simulink model "Appl_VentAdj_CtrlModel"  (R2018b)
settings: configuration reference "CodeConfig_10_ms" (kept outside this file)
undefined symbols (not defined in the file): D_VENT_LVL_1_PRECENT, D_VENT_LVL_2_PRECENT, D_VENT_LVL_3_PRECENT, FALSE, TRUE
libraries: DareLib x72, simulink x1
(part 3 of 4)

== stateflow chart Appl_VentAdj_CtrlModel/LogicCtrl/LocalAdjustCtrl/LimitDeal/TimeoutFunction1/Timeout ==
  state Ts = D_HAL_GET_CUR_MS_TS [function]
  state OutTs = TimeDiffTs(lastTs,Ts) [function]
  state TimeCountStatus
    state TimeoutSts
      en:
      Level = InLevel;
      du:
      Level = InLevel;
      ex:
      Timer = 0;
    state Init
      en:
      Level = InLevel;
      Timer = D_HAL_GET_CUR_MS_TS();
      du:
      Level = InLevel;
      ex:
      Timer = D_HAL_GET_CUR_MS_TS();
    (default) -> Init
    Init -> TimeoutSts [order 1] : [TimeDiffTs(Timer,D_HAL_GET_CUR_MS_TS()) >= MaxTime]
        | /TimeoutFlag = TRUE;
    TimeoutSts -> Init : [hasChangedFrom(InLevel,enVentLvlSts.EN_VENT_LVL_OFF)]
    Init -> Init [order 2] : [hasChangedFrom(InLevel,enVentLvlSts.EN_VENT_LVL_OFF)]
  state Default
    en:
    Level = InLevel;
    du:
    Level = InLevel;
  (default) -> Default
  Default -> TimeCountStatus : /*有超时配置
      | && 启动加热&&有时间值 */
      | [TRUE == TimeoutPrm ...
      | && enVentLvlSts.EN_VENT_LVL_OFF != InLevel ...
      | && 0 != MaxTime]
  TimeCountStatus -> Default : /*无超时配置*/
      | [TRUE != TimeoutPrm || 0 == MaxTime]
      | /TimeoutFlag = FALSE;
  data: Ts function_output; lastTs function_input; Ts function_input; OutTs function_output; TimeoutPrm input uint8; TimeoutFlag output uint8; FALSE parameter; TRUE parameter; InLevel input Enum: enVentLvlSts; MaxTime input uint32; Timer local uint32; Level output Enum: enVentLvlSts

== stateflow chart Appl_VentAdj_CtrlModel/UpDataInputInfo/InputSignalProcess/HeatMessage/HeatMessage ==
  state VenSts = OppositeMessageDeal(CarTypeCfg,RemoteModeFlag,HMI_Message,Tbox_Message,HeatCfg) [function]
  state VenSts = OppositeMessageDeal1(CarTypeCfg,RemoteModeFlag,HMI_Message,Tbox_Message,HeatCfg) [function]
  state VenSts = OppositeMessageDeal2(CarTypeCfg,RemoteModeFlag,HMI_Message,Tbox_Message,HeatCfg) [function]
  state run
    du:
    DriverHeatValid = OppositeMessageDeal(VentAdj_CarType,VentAdj_RemoteModeFlag,VentAdj_Driver_HMI_HeatMsg,VentAdj_Driver_Tbox_HeatMsg,VentAdj_DrHeatFlg);
    PassengerHeatValid = OppositeMessageDeal1(VentAdj_CarType,VentAdj_RemoteModeFlag,VentAdj_Passenger_HMI_HeatMsg,VentAdj_Passenger_Tbox_HeatMsg,VentAdj_PaHeatFlg);
    ThirdHeatValid = OppositeMessageDeal2(VentAdj_CarType,VentAdj_RemoteModeFlag,VentAdj_Third_HMI_HeatMsg,VentAdj_Third_Tbox_HeatMsg,VentAdj_3rdHeatFlg);
  (default) -> run
  data: CarTypeCfg function_input; RemoteModeFlag function_input; HMI_Message function_input; Tbox_Message function_input; VenSts function_output; HeatCfg function_input; CarTypeCfg function_input; RemoteModeFlag function_input; HMI_Message function_input; Tbox_Message function_input; VenSts function_output; HeatCfg function_input; CarTypeCfg function_input; RemoteModeFlag function_input; HMI_Message function_input; Tbox_Message function_input; VenSts function_output; HeatCfg function_input; DriverHeatValid output uint8; PassengerHeatValid output uint8; ThirdHeatValid output uint8; VentAdj_CarType input; VentAdj_Driver_HMI_HeatMsg input; VentAdj_Driver_Tbox_HeatMsg input; VentAdj_Passenger_HMI_HeatMsg input; VentAdj_Passenger_Tbox_HeatMsg input; VentAdj_Third_HMI_HeatMsg input; VentAdj_Third_Tbox_HeatMsg input; VentAdj_RemoteModeFlag input; VentAdj_DrHeatFlg input; VentAdj_PaHeatFlg input; VentAdj_3rdHeatFlg input

== stateflow chart Appl_VentAdj_CtrlModel/UpDataInputInfo/InputSignalProcess/HeatMessage/HeatMessage/OppositeMessageDeal1/OppositeMessageDeal ==
  state HMIMessageDeal [parallel]
    settings: executionOrder=1
    state HMIValid
      en:
      TempHMI = TRUE;
    state HMIInit
      en:
      TempHMI = FALSE;
    (default) -> HMIInit
    HMIInit -> HMIValid : /*档位请求有效*/
        | [(enProjectType.EN_PROJECT_BM400 != CarTypeCfg && (0x1 == HMI_Message || 0x2 == HMI_Message || 0x3 == HMI_Message || 0x5 == HMI_Message)) ...
        | || (enProjectType.EN_PROJECT_BM400 == CarTypeCfg && (0x2 == HMI_Message || 0x3 == HMI_Message || 0x4 == HMI_Message))]
    HMIValid -> HMIInit : /*HMI报文关闭*/
        | [(enProjectType.EN_PROJECT_BM400 != CarTypeCfg && 0x1 != HMI_Message && 0x2 != HMI_Message && 0x3 != HMI_Message&& 0x5 != HMI_Message) ...
        | || (enProjectType.EN_PROJECT_BM400 == CarTypeCfg && 0x2 != HMI_Message && 0x3 != HMI_Message && 0x4 != HMI_Message)]
  state TboxMessageDeal [parallel]
    settings: executionOrder=2
    state TboxValid
      en:
      TempTbox = TRUE;
    state TboxInit
      en:
      TempTbox = FALSE;
    (default) -> TboxMessageDeal.TboxInit
    TboxMessageDeal.TboxInit -> TboxMessageDeal.TboxValid : /*档位请求有效*/
        | [(TRUE == RemoteModeFlag) && (0x1 == Tbox_Message ...
        | || 0x2 == Tbox_Message ...
        | || 0x3 == Tbox_Message)]
    TboxMessageDeal.TboxValid -> TboxMessageDeal.TboxInit : /*Tbox报文关闭*/
        | [0x0 == Tbox_Message || FALSE == RemoteModeFlag]
  state VenStatus [parallel]
    settings: executionOrder=3
    state TboxValid
      en:
      VenSts = TRUE;
    state TboxInit
      en:
      VenSts = FALSE;
    (default) -> VenStatus.TboxInit
    VenStatus.TboxInit -> VenStatus.TboxValid : /* 档位请求有效 且加热配置 */
        | [(TRUE == TempHMI ...
        | || TRUE == TempTbox) && HeatCfg == TRUE]
    VenStatus.TboxValid -> VenStatus.TboxInit : /* 档位请求无效 或加热无配置 */
        | [(FALSE == TempHMI ...
        | && FALSE == TempTbox) || HeatCfg == FALSE]
  data: CarTypeCfg input Enum: enProjectType; RemoteModeFlag input uint8; HMI_Message input uint8; Tbox_Message input uint8; VenSts output uint8; TempHMI local uint8; TRUE parameter; FALSE parameter; TempTbox local uint8; HeatCfg input uint8

== stateflow chart Appl_VentAdj_CtrlModel/LogicCtrl/LocalAdjustCtrl/LimitDeal/DiagnoseFunction1/Diagnose ==
  state Diagnose
    (default) -> (junction 3)
    Diagnose -> (junction 3)
    (junction 3) -> (junction 6)
    (junction 6) -> (junction 8) [order 1] : /* 无诊断指令 */
        | [0 == DiagCommand || DiagCommand > (enVentLvlSts.EN_VENT_LVL_3 + 1)]
    (junction 6) -> (junction 14) [order 2] : {Level = DiagCommand - 1;
        | Type = enVentType.EN_VENT_TYPE_DIAG;}
    (junction 8) -> (junction 10) : {Level = InLevel;
        | Type = CurrentType;}
    (junction 10) -> (junction 14)
    (junction 14) -> (junction 17)
  (default) -> Diagnose
  data: DiagCommand input uint8; InLevel input Enum: enVentLvlSts; CurrentType input Enum: enVentType; Level output Enum: enVentLvlSts; Type output Enum: enVentType

== stateflow chart Appl_VentAdj_CtrlModel/LogicCtrl/LocalAdjustCtrl/LimitDeal/DiagnoseFunction2/Diagnose ==
  state Diagnose
    (default) -> (junction 3)
    Diagnose -> (junction 3)
    (junction 3) -> (junction 6)
    (junction 6) -> (junction 8) [order 1] : /* 无诊断指令 */
        | [0 == DiagCommand || DiagCommand > (enVentLvlSts.EN_VENT_LVL_3 + 1)]
    (junction 6) -> (junction 14) [order 2] : {Level = DiagCommand - 1;
        | Type = enVentType.EN_VENT_TYPE_DIAG;}
    (junction 8) -> (junction 10) : {Level = InLevel;
        | Type = CurrentType;}
    (junction 10) -> (junction 14)
    (junction 14) -> (junction 17)
  (default) -> Diagnose
  data: DiagCommand input uint8; InLevel input Enum: enVentLvlSts; CurrentType input Enum: enVentType; Level output Enum: enVentLvlSts; Type output Enum: enVentType

== stateflow chart Appl_VentAdj_CtrlModel/LogicCtrl/LocalAdjustCtrl/LimitDeal/StopFunction1/StopFunction ==
  state ValidSts
    en:
    StopReason = enVentStopReason.EN_VENT_STOP_R_TIME;
    du:
    StopReason = enVentStopReason.EN_VENT_STOP_R_TIME;
  state Default
    en:
    du:
    StopReason = ComStop;
    du:
    StopReason = ComStop;
  (default) -> Default
  Default -> ValidSts : /*无通用限制
      | &&超时限制有效*/
      | [enVentStopReason.EN_VENT_STOP_R_NONE == ComStop ...
      | && TRUE  == Timeout]
  ValidSts -> Default : /*无超时限制*/
      | [FALSE  == Timeout]
  data: FALSE parameter; StopReason output Enum: enVentStopReason; Timeout input uint8; ComStop input Enum: enVentStopReason; TRUE parameter

== stateflow chart Appl_VentAdj_CtrlModel/LogicCtrl/LocalAdjustCtrl/LimitDeal/StopFunction2/StopFunction ==
  state ValidSts
    en:
    StopReason = enVentStopReason.EN_VENT_STOP_R_TIME;
    du:
    StopReason = enVentStopReason.EN_VENT_STOP_R_TIME;
  state Default
    en:
    du:
    StopReason = ComStop;
    du:
    StopReason = ComStop;
  (default) -> Default
  Default -> ValidSts : /*无通用限制
      | &&超时限制有效*/
      | [enVentStopReason.EN_VENT_STOP_R_NONE == ComStop ...
      | && TRUE  == Timeout]
  ValidSts -> Default : /*无超时限制*/
      | [FALSE  == Timeout]
  data: FALSE parameter; StopReason output Enum: enVentStopReason; Timeout input uint8; ComStop input Enum: enVentStopReason; TRUE parameter

== stateflow chart Appl_VentAdj_CtrlModel/LogicCtrl/LocalAdjustCtrl/LimitDeal/StopFunction/StopFunction ==
  state ValidSts
    en:
    StopReason = enVentStopReason.EN_VENT_STOP_R_TIME;
    du:
    StopReason = enVentStopReason.EN_VENT_STOP_R_TIME;
  state Default
    en:
    du:
    StopReason = ComStop;
    du:
    StopReason = ComStop;
  (default) -> Default
  Default -> ValidSts : /*无通用限制
      | &&超时限制有效*/
      | [enVentStopReason.EN_VENT_STOP_R_NONE == ComStop ...
      | && TRUE  == Timeout]
  ValidSts -> Default : /*无超时限制*/
      | [FALSE  == Timeout]
  data: FALSE parameter; StopReason output Enum: enVentStopReason; Timeout input uint8; ComStop input Enum: enVentStopReason; TRUE parameter

== stateflow chart Appl_VentAdj_CtrlModel/LogicCtrl/LocalAdjustCtrl/LimitDeal/DiagnoseFunction/Diagnose ==
  state Diagnose
    (default) -> (junction 3)
    Diagnose -> (junction 3)
    (junction 3) -> (junction 6)
    (junction 6) -> (junction 8) [order 1] : /* 无诊断指令 */
        | [0 == DiagCommand || DiagCommand > (enVentLvlSts.EN_VENT_LVL_3 + 1)]
    (junction 6) -> (junction 14) [order 2] : {Level = DiagCommand - 1;
        | Type = enVentType.EN_VENT_TYPE_DIAG;}
    (junction 8) -> (junction 10) : {Level = InLevel;
        | Type = CurrentType;}
    (junction 10) -> (junction 14)
    (junction 14) -> (junction 17)
  (default) -> Diagnose
  data: DiagCommand input uint8; InLevel input Enum: enVentLvlSts; CurrentType input Enum: enVentType; Level output Enum: enVentLvlSts; Type output Enum: enVentType

== stateflow chart Appl_VentAdj_CtrlModel/LogicCtrl/LocalAdjustCtrl/OutputDeal ==
  state CANOutputDeal [parallel]
    settings: executionOrder=1
    state ProjectP20
      en:
      /*Initial Value(Hex)初始值:0x0*/
      OutDrCANVentLevel = 0;
      OutPaCANVentLevel = 0;
      Out3rdCANVentLevel = 0;
      state Drv [parallel]
        settings: executionOrder=1
        state Run
          en:
          OutDrCANVentLevel = DiagDrVentLevel;
          LocalDrRunState = TRUE;
          du:
          OutDrCANVentLevel = DiagDrVentLevel;
          LocalDrRunState = TRUE;
        state Init
          en:
          LocalDrRunState = FALSE;
        (default) -> CANOutputDeal.ProjectP20.Drv.Init
        CANOutputDeal.ProjectP20.Drv.Init -> CANOutputDeal.ProjectP20.Drv.Run : /* 主驾通风指令 */
            | [enVentLvlSts.EN_VENT_LVL_OFF != DiagDrVentLevel]
        CANOutputDeal.ProjectP20.Drv.Run -> CANOutputDeal.ProjectP20.Drv.Init : /* 主驾通风无指令 */
            | [enVentLvlSts.EN_VENT_LVL_OFF == DiagDrVentLevel]
      state Pas [parallel]
        settings: executionOrder=2
        state Run
          en:
          OutPaCANVentLevel = DiagPaVentLevel;
          LocalPaRunState = TRUE;
          du:
          OutPaCANVentLevel = DiagPaVentLevel;
          LocalPaRunState = TRUE;
        state Init
          en:
          LocalPaRunState = FALSE;
        (default) -> CANOutputDeal.ProjectP20.Pas.Init
        CANOutputDeal.ProjectP20.Pas.Run -> CANOutputDeal.ProjectP20.Pas.Init : /* 副驾通风无指令 */
            | [enVentLvlSts.EN_VENT_LVL_OFF == DiagPaVentLevel]
        CANOutputDeal.ProjectP20.Pas.Init -> CANOutputDeal.ProjectP20.Pas.Run : /* 副驾通风指令 */
            | [enVentLvlSts.EN_VENT_LVL_OFF != DiagPaVentLevel]
      state Treble [parallel]
        settings: executionOrder=3
        state Init
          en:
          Local3rdRunState = FALSE;
        state Run
          en:
          Out3rdCANVentLevel = Diag3rdVentLevel;
          Local3rdRunState = TRUE;
          du:
          Out3rdCANVentLevel = Diag3rdVentLevel;
          Local3rdRunState = TRUE;
        (default) -> CANOutputDeal.ProjectP20.Treble.Init
        CANOutputDeal.ProjectP20.Treble.Init -> CANOutputDeal.ProjectP20.Treble.Run : /* 三排通风无指令 */
            | [enVentLvlSts.EN_VENT_LVL_OFF != Diag3rdVentLevel]
        CANOutputDeal.ProjectP20.Treble.Run -> CANOutputDeal.ProjectP20.Treble.Init : /* 三排通风无指令 */
            | [enVentLvlSts.EN_VENT_LVL_OFF == Diag3rdVentLevel]
    state Default
      en:
      OutDrCANVentLevel = DiagDrVentLevel;
      OutPaCANVentLevel = DiagPaVentLevel;
      Out3rdCANVentLevel = Diag3rdVentLevel;
      OutDrRunState = FALSE;
      OutPaRunState = FALSE;
      Out3rdRunState = FALSE;
      LocalDrRunState = FALSE;
      LocalDrRunState = FALSE;
      LocalDrRunState = FALSE;
      du:
      OutDrCANVentLevel = DiagDrVentLevel;
      OutPaCANVentLevel = DiagPaVentLevel;
      Out3rdCANVentLevel = Diag3rdVentLevel;
      OutDrRunState = FALSE;
      OutPaRunState = FALSE;
      Out3rdRunState = FALSE;
      LocalDrRunState = FALSE;
      LocalDrRunState = FALSE;
      LocalDrRunState = FALSE;
    (default) -> Default
    Default -> ProjectP20 : /* P20的车型 */
        | [enProjectType.EN_PROJECT_P20 == CarTypeCfg]
    ProjectP20 -> Default : /* 非P20车型 */
        | [enProjectType.EN_PROJECT_P20 != CarTypeCfg]
  state DrvErr [parallel]
    settings: executionOrder=2
    state FalseSts
      en:
      OutDrRunState = LocalDrRunState;
      du:
      OutDrRunState = LocalDrRunState;
    state SuccSts
      en:
      OutDrRunState = 2;
      du:
      OutDrRunState = 2;
    (default) -> DrvErr.FalseSts
    DrvErr.FalseSts -> DrvErr.SuccSts : /* 无指令 且存在故障 */
        | [LocalDrRunState == FALSE ...
        | && VentAdj_DriverCmdFaultSts4DTC != FALSE]
    DrvErr.SuccSts -> DrvErr.FalseSts : /*无故障 或RUN状态 */
        | [LocalDrRunState == TRUE ...
        | || VentAdj_DriverCmdFaultSts4DTC ==  FALSE]
  state AcquireDuty [parallel]
    en:
    DrAimDuty = DutyFunction(DiagDrVentLevel);
    PaAimDuty = DutyFunction(DiagPaVentLevel);
    ThirdAimDuty = DutyFunction(Diag3rdVentLevel);
    du:
    DrAimDuty = DutyFunction(DiagDrVentLevel);
    PaAimDuty = DutyFunction(DiagPaVentLevel);
    ThirdAimDuty = DutyFunction(Diag3rdVentLevel);
    settings: executionOrder=5
  state AimDuty = DutyFunction(AimLevel) [function]
  state PasErr [parallel]
    settings: executionOrder=3
    state FalseSts
      en:
      OutPaRunState = LocalPaRunState;
      du:
      OutPaRunState = LocalPaRunState;
    state SuccSts
      en:
      OutPaRunState = 2;
      du:
      OutPaRunState = 2;
    (default) -> PasErr.FalseSts
    PasErr.FalseSts -> PasErr.SuccSts : /* 无指令 且存在故障 */
        | [LocalPaRunState == FALSE ...
        | && VentAdj_PasCmdFaultSts4DTC != FALSE]
    PasErr.SuccSts -> PasErr.FalseSts : /*无故障 或RUN状态 */
        | [LocalPaRunState == TRUE ...
        | || VentAdj_PasCmdFaultSts4DTC == FALSE]
  state TrebleErr [parallel]
    settings: executionOrder=4
    state FalseSts
      en:
      Out3rdRunState = Local3rdRunState;
      du:
      Out3rdRunState = Local3rdRunState;
    state SuccSts
      en:
      Out3rdRunState = 2;
      du:
      Out3rdRunState = 2;
    (default) -> TrebleErr.FalseSts
    TrebleErr.FalseSts -> TrebleErr.SuccSts : /* 无指令 且存在故障 */
        | [Local3rdRunState == FALSE ...
        | && VentAdj_ThirdCmdFaultSts4DTC != FALSE]
    TrebleErr.SuccSts -> TrebleErr.FalseSts : /*无故障 或RUN状态 */
        | [Local3rdRunState == TRUE ...
        | || VentAdj_ThirdCmdFaultSts4DTC == FALSE]
  data: AimLevel function_input; AimDuty function_output; OutDrCANVentLevel output Enum: enVentLvlSts; OutPaCANVentLevel output Enum: enVentLvlSts; Out3rdCANVentLevel output Enum: enVentLvlSts; CarTypeCfg input; DiagDrVentLevel input; DiagPaVentLevel input; Diag3rdVentLevel input; FALSE parameter; OutDrRunState output uint8; OutPaRunState output uint8; Out3rdRunState output uint8; TRUE parameter; DrAimDuty output uint8; PaAimDuty output uint8; ThirdAimDuty output uint8; LocalDrRunState local uint8; LocalPaRunState local uint8; Local3rdRunState local uint8; VentAdj_DriverCmdFaultSts4DTC input; VentAdj_PasCmdFaultSts4DTC input; VentAdj_ThirdCmdFaultSts4DTC input

== stateflow chart Appl_VentAdj_CtrlModel/LogicCtrl/LocalAdjustCtrl/OutputDeal/DutyFunction/Duty ==
  (default) -> (junction 3)
  (junction 3) -> (junction 5) : {AimDuty = 100;}
  (junction 5) -> (junction 7) [order 1] : /* 通风1档 */
      | [enVentLvlSts.EN_VENT_LVL_1 == AimLevel]
  (junction 5) -> (junction 11) [order 2]
  (junction 7) -> (junction 9) : {AimDuty = D_VENT_LVL_1_PRECENT;}
  (junction 9) -> (junction 11)
  (junction 11) -> (junction 14)
  (junction 14) -> (junction 16) [order 1] : /* 通风2档 */
      | [enVentLvlSts.EN_VENT_LVL_2 == AimLevel]
  (junction 14) -> (junction 20) [order 2]
  (junction 16) -> (junction 18) : {AimDuty = D_VENT_LVL_2_PRECENT;}
  (junction 18) -> (junction 20)
  (junction 20) -> (junction 23)
  (junction 23) -> (junction 25) [order 1] : /* 通风3档 */
      | [enVentLvlSts.EN_VENT_LVL_3 == AimLevel]
  (junction 23) -> (junction 29) [order 2]
  (junction 25) -> (junction 27) : {AimDuty = D_VENT_LVL_3_PRECENT;}
  (junction 27) -> (junction 29)
  (junction 29) -> (junction 35)
  data: AimDuty output uint8; AimLevel input Enum: enVentLvlSts; D_VENT_LVL_1_PRECENT parameter; D_VENT_LVL_2_PRECENT parameter; D_VENT_LVL_3_PRECENT parameter

== stateflow chart Appl_VentAdj_CtrlModel/LogicCtrl/LocalAdjustCtrl/VentLevelDeal/VentRunTypeFunction/VentRunType ==
  (default) -> (junction 82)
  (junction 82) -> (junction 84) : {OutLevel = PreLevel;}
  (junction 84) -> (junction 86) [order 1] : /* 有效档位 */
      | [InLevel <= enVentLvlSts.EN_VENT_LVL_3]
  (junction 84) -> (junction 90) [order 2]
  (junction 86) -> (junction 88) : {RunType = InType;
      | OutLevel = InLevel;}
  (junction 88) -> (junction 90)
  (junction 90) -> (junction 93)
  (junction 93) -> (junction 95) [order 1] : /* 通风档位关闭 */
      | [InLevel == enVentLvlSts.EN_VENT_LVL_OFF]
  (junction 93) -> (junction 99) [order 2]
  (junction 95) -> (junction 97) : {RunType = enVentType.EN_VENT_TYPE_NONE;}
  (junction 97) -> (junction 99)
  (junction 99) -> (junction 102)
  data: InLevel input uint8; PreLevel input Enum: enVentLvlSts; InType input Enum: enVentType; RunType output Enum: enVentType; OutLevel output Enum: enVentLvlSts

== stateflow chart Appl_VentAdj_CtrlModel/LogicCtrl/LocalAdjustCtrl/LimitDeal/TimeoutFunction1/Timeout/TimeDiffTs/Chart ==
  (default) -> (junction 3)
  (junction 3) -> (junction 5)
  (junction 5) -> (junction 7) [order 1] : /* 入参比当前大 */
      | [lastTs > Ts]
  (junction 5) -> (junction 13) [order 2] : {OutTs = Ts - lastTs;}
  (junction 7) -> (junction 11) : {OutTs = 0xFFFFFFFF - lastTs + Ts +1;}
  (junction 11) -> (junction 13)
  (junction 13) -> (junction 17)
  data: lastTs input uint32; Ts input uint32; OutTs output uint32

== stateflow chart Appl_VentAdj_CtrlModel/UpDataInputInfo/InputSignalProcess/HeatMessage/HeatMessage/OppositeMessageDeal/OppositeMessageDeal ==
  state HMIMessageDeal [parallel]
    settings: executionOrder=1
    state HMIValid
      en:
      TempHMI = TRUE;
    state HMIInit
      en:
      TempHMI = FALSE;
    (default) -> HMIInit
    HMIInit -> HMIValid : /*档位请求有效*/
        | [(enProjectType.EN_PROJECT_BM400 != CarTypeCfg && (0x1 == HMI_Message || 0x2 == HMI_Message || 0x3 == HMI_Message || 0x5 == HMI_Message)) ...
        | || (enProjectType.EN_PROJECT_BM400 == CarTypeCfg && (0x2 == HMI_Message || 0x3 == HMI_Message || 0x4 == HMI_Message))]
    HMIValid -> HMIInit : /*HMI报文关闭*/
        | [(enProjectType.EN_PROJECT_BM400 != CarTypeCfg && 0x1 != HMI_Message && 0x2 != HMI_Message && 0x3 != HMI_Message&& 0x5 != HMI_Message) ...
        | || (enProjectType.EN_PROJECT_BM400 == CarTypeCfg && 0x2 != HMI_Message && 0x3 != HMI_Message && 0x4 != HMI_Message)]
  state TboxMessageDeal [parallel]
    settings: executionOrder=2
    state TboxValid
      en:
      TempTbox = TRUE;
    state TboxInit
      en:
      TempTbox = FALSE;
    (default) -> TboxMessageDeal.TboxInit
    TboxMessageDeal.TboxInit -> TboxMessageDeal.TboxValid : /*档位请求有效*/
        | [(TRUE == RemoteModeFlag) && (0x1 == Tbox_Message ...
        | || 0x2 == Tbox_Message ...
        | || 0x3 == Tbox_Message)]
    TboxMessageDeal.TboxValid -> TboxMessageDeal.TboxInit : /*Tbox报文关闭*/
        | [0x0 == Tbox_Message || FALSE == RemoteModeFlag]
  state VenStatus [parallel]
    settings: executionOrder=3
    state TboxValid
      en:
      VenSts = TRUE;
    state TboxInit
      en:
      VenSts = FALSE;
    (default) -> VenStatus.TboxInit
    VenStatus.TboxInit -> VenStatus.TboxValid : /* 档位请求有效 且加热配置 */
        | [(TRUE == TempHMI ...
        | || TRUE == TempTbox) && HeatCfg == TRUE]
    VenStatus.TboxValid -> VenStatus.TboxInit : /* 档位请求无效 或加热无配置 */
        | [(FALSE == TempHMI ...
        | && FALSE == TempTbox) || HeatCfg == FALSE]
  data: CarTypeCfg input Enum: enProjectType; RemoteModeFlag input uint8; HMI_Message input uint8; Tbox_Message input uint8; VenSts output uint8; TempHMI local uint8; TRUE parameter; FALSE parameter; TempTbox local uint8; HeatCfg input uint8

== stateflow chart Appl_VentAdj_CtrlModel/LogicCtrl/LocalAdjustCtrl/LimitDeal/TimeoutFunction2/Timeout ==
  state Ts = D_HAL_GET_CUR_MS_TS [function]
  state OutTs = TimeDiffTs(lastTs,Ts) [function]
  state TimeCountStatus
    state TimeoutSts
      en:
      Level = InLevel;
      du:
      Level = InLevel;
      ex:
      Timer = 0;
    state Init
      en:
      Level = InLevel;
      Timer = D_HAL_GET_CUR_MS_TS();
      du:
      Level = InLevel;
      ex:
      Timer = D_HAL_GET_CUR_MS_TS();
    (default) -> Init
    Init -> TimeoutSts [order 1] : [TimeDiffTs(Timer,D_HAL_GET_CUR_MS_TS()) >= MaxTime]
        | /TimeoutFlag = TRUE;
    TimeoutSts -> Init : [hasChangedFrom(InLevel,enVentLvlSts.EN_VENT_LVL_OFF)]
    Init -> Init [order 2] : [hasChangedFrom(InLevel,enVentLvlSts.EN_VENT_LVL_OFF)]
  state Default
    en:
    Level = InLevel;
    du:
    Level = InLevel;
  (default) -> Default
  Default -> TimeCountStatus : /*有超时配置
      | && 启动加热&&有时间值 */
      | [TRUE == TimeoutPrm ...
      | && enVentLvlSts.EN_VENT_LVL_OFF != InLevel ...
      | && 0 != MaxTime]
  TimeCountStatus -> Default : /*无超时配置*/
      | [TRUE != TimeoutPrm || 0 == MaxTime]
      | /TimeoutFlag = FALSE;
  data: Ts function_output; lastTs function_input; Ts function_input; OutTs function_output; TimeoutPrm input uint8; TimeoutFlag output uint8; FALSE parameter; TRUE parameter; InLevel input Enum: enVentLvlSts; MaxTime input uint32; Timer local uint32; Level output Enum: enVentLvlSts

== stateflow chart Appl_VentAdj_CtrlModel/LogicCtrl/LocalAdjustCtrl/LimitDeal/TimeoutFunction2/Timeout/TimeDiffTs/Chart ==
  (default) -> (junction 3)
  (junction 3) -> (junction 5)
  (junction 5) -> (junction 7) [order 1] : /* 入参比当前大 */
      | [lastTs > Ts]
  (junction 5) -> (junction 13) [order 2] : {OutTs = Ts - lastTs;}
  (junction 7) -> (junction 11) : {OutTs = 0xFFFFFFFF - lastTs + Ts +1;}
  (junction 11) -> (junction 13)
  (junction 13) -> (junction 17)
  data: lastTs input uint32; Ts input uint32; OutTs output uint32

== stateflow chart Appl_VentAdj_CtrlModel/LogicCtrl/LocalAdjustCtrl/LimitDeal/LevelLimitFunction/LevelLimit ==
  state Default
    en:
    Level = enVentLvlSts.EN_VENT_LVL_OFF;
  state Run
    en:
    Level = OriginalLevel;
    du:
    Level = OriginalLevel;
  state ForbidStatus
    en:
    Level = enVentLvlSts.EN_VENT_LVL_OFF;
    ex:
    StopReason = enVentStopReason.EN_VENT_STOP_R_NONE;
    (default) -> (junction 74)
    ForbidStatus -> (junction 74) [order 1]
    (junction 74) -> (junction 46) [order 1] : /*存在故障*/
        | [enVentCmdFault.EN_VENT_FAULT_NONE != Error]
    (junction 74) -> (junction 71) [order 2]
    (junction 46) -> (junction 60) : {StopReason = enVentStopReason.EN_VENT_STOP_R_FAULT;}
    (junction 60) -> (junction 71)
    (junction 71) -> (junction 70)
    (junction 70) -> (junction 43) [order 1] : /*互斥命令有效*/
        | [TRUE == OppositeCmd]
    (junction 70) -> (junction 54) [order 2]
    (junction 43) -> (junction 49) : {StopReason = enVentStopReason.EN_VENT_STOP_R_CMD;}
    (junction 49) -> (junction 54)
    (junction 54) -> (junction 59)
    (junction 59) -> (junction 78) [order 1] : /*恢复出厂*/
        | [TRUE == Vent_RecoverDefaultFlag]
    (junction 59) -> (junction 57) [order 2]
    (junction 78) -> (junction 42) : {StopReason = enVentStopReason.EN_VENT_STOP_R_FACTORY;}
    (junction 42) -> (junction 57)
    (junction 57) -> (junction 51)
    (junction 51) -> (junction 48) [order 1] : /*BM400掉线禁能*/
        | [TRUE == Vent_CanMessageLostFlag && enProjectType.EN_PROJECT_BM400 == CarType]
    (junction 51) -> (junction 40) [order 2]
    (junction 48) -> (junction 65) : {StopReason = enVentStopReason.EN_VENT_STOP_R_LOSS;}
    (junction 65) -> (junction 40)
    (junction 40) -> (junction 68)
  (default) -> Default
  ForbidStatus -> Default [order 1] : /*无用户请求，可准备下一轮禁能原因检测*/
      | [enVentLvlSts.EN_VENT_LVL_OFF == OriginalLevel]
  Default -> ForbidStatus : /*请求工作*/
      | [enVentLvlSts.EN_VENT_LVL_OFF != OriginalLevel]
  Run -> ForbidStatus [commented out] : /*非正常电压模式*/
      | [enFinalPowerMode.EN_NORMAL_VOLT != VoltMode]
      | /StopReason = enVentStopReason.EN_VENT_STOP_R_VOL;
  Run -> ForbidStatus [order 1] : /*存在故障*/
      | [enVentCmdFault.EN_VENT_FAULT_NONE != Error]
      | /StopReason = enVentStopReason.EN_VENT_STOP_R_FAULT;
  Run -> ForbidStatus [order 2] : /*互斥命令有效*/
      | [TRUE == OppositeCmd]
      | /StopReason = enVentStopReason.EN_VENT_STOP_R_CMD;
  Run -> ForbidStatus [order 3] : /*恢复出厂*/
      | [TRUE == Vent_RecoverDefaultFlag]
      | /StopReason = enVentStopReason.EN_VENT_STOP_R_FACTORY;
  Run -> ForbidStatus [order 4] : /*BM400掉线禁能*/
      | [TRUE == Vent_CanMessageLostFlag && enProjectType.EN_PROJECT_BM400 == CarType]
      | /StopReason = enVentStopReason.EN_VENT_STOP_R_LOSS;
  ForbidStatus -> Run [order 2] : /*无故障
      | && 互斥命令无效
      | && 无恢复出厂命令
      | && （BM400控制报文在线 || 非BM400车型）*/
      | [enVentCmdFault.EN_VENT_FAULT_NONE == Error ...
      | && TRUE != OppositeCmd ...
      | && TRUE != Vent_RecoverDefaultFlag ...
      | && ((FALSE == Vent_CanMessageLostFlag && enProjectType.EN_PROJECT_BM400 == CarType) ...
      | || (enProjectType.EN_PROJECT_BM400 != CarType))]
  data: Level output Enum: enVentLvlSts; StopReason output Enum: enVentStopReason; OriginalLevel input Enum: enVentLvlSts; Error input uint8; CarType input Enum: enProjectType; TRUE parameter; OppositeCmd input uint8; Vent_CanMessageLostFlag input uint8; Vent_RecoverDefaultFlag input uint8; FALSE parameter

== stateflow chart Appl_VentAdj_CtrlModel/LogicCtrl/LocalAdjustCtrl/LimitDeal/LevelLimitFunction2/LevelLimit ==
  state Default
    en:
    Level = enVentLvlSts.EN_VENT_LVL_OFF;
  state Run
    en:
    Level = OriginalLevel;
    du:
    Level = OriginalLevel;
  state ForbidStatus
    en:
    Level = enVentLvlSts.EN_VENT_LVL_OFF;
    ex:
    StopReason = enVentStopReason.EN_VENT_STOP_R_NONE;
    (default) -> (junction 74)
    ForbidStatus -> (junction 74) [order 1]
    (junction 74) -> (junction 46) [order 1] : /*存在故障*/
        | [enVentCmdFault.EN_VENT_FAULT_NONE != Error]
    (junction 74) -> (junction 71) [order 2]
    (junction 46) -> (junction 60) : {StopReason = enVentStopReason.EN_VENT_STOP_R_FAULT;}
    (junction 60) -> (junction 71)
    (junction 71) -> (junction 70)
    (junction 70) -> (junction 43) [order 1] : /*互斥命令有效*/
        | [TRUE == OppositeCmd]
    (junction 70) -> (junction 54) [order 2]
    (junction 43) -> (junction 49) : {StopReason = enVentStopReason.EN_VENT_STOP_R_CMD;}
    (junction 49) -> (junction 54)
    (junction 54) -> (junction 59)
    (junction 59) -> (junction 78) [order 1] : /*恢复出厂*/
        | [TRUE == Vent_RecoverDefaultFlag]
    (junction 59) -> (junction 57) [order 2]
    (junction 78) -> (junction 42) : {StopReason = enVentStopReason.EN_VENT_STOP_R_FACTORY;}
    (junction 42) -> (junction 57)
    (junction 57) -> (junction 51)
    (junction 51) -> (junction 48) [order 1] : /*BM400掉线禁能*/
        | [TRUE == Vent_CanMessageLostFlag && enProjectType.EN_PROJECT_BM400 == CarType]
    (junction 51) -> (junction 40) [order 2]
    (junction 48) -> (junction 65) : {StopReason = enVentStopReason.EN_VENT_STOP_R_LOSS;}
    (junction 65) -> (junction 40)
    (junction 40) -> (junction 68)
  (default) -> Default
  ForbidStatus -> Default [order 1] : /*无用户请求，可准备下一轮禁能原因检测*/
      | [enVentLvlSts.EN_VENT_LVL_OFF == OriginalLevel]
  Default -> ForbidStatus : /*请求工作*/
      | [enVentLvlSts.EN_VENT_LVL_OFF != OriginalLevel]
  Run -> ForbidStatus [commented out] : /*非正常电压模式*/
      | [enFinalPowerMode.EN_NORMAL_VOLT != VoltMode]
      | /StopReason = enVentStopReason.EN_VENT_STOP_R_VOL;
  Run -> ForbidStatus [order 1] : /*存在故障*/
      | [enVentCmdFault.EN_VENT_FAULT_NONE != Error]
      | /StopReason = enVentStopReason.EN_VENT_STOP_R_FAULT;
  Run -> ForbidStatus [order 2] : /*互斥命令有效*/
      | [TRUE == OppositeCmd]
      | /StopReason = enVentStopReason.EN_VENT_STOP_R_CMD;
  Run -> ForbidStatus [order 3] : /*恢复出厂*/
      | [TRUE == Vent_RecoverDefaultFlag]
      | /StopReason = enVentStopReason.EN_VENT_STOP_R_FACTORY;
  Run -> ForbidStatus [order 4] : /*BM400掉线禁能*/
      | [TRUE == Vent_CanMessageLostFlag && enProjectType.EN_PROJECT_BM400 == CarType]
      | /StopReason = enVentStopReason.EN_VENT_STOP_R_LOSS;
  ForbidStatus -> Run [order 2] : /*无故障
      | && 互斥命令无效
      | && 无恢复出厂命令
      | && （BM400控制报文在线 || 非BM400车型）*/
      | [enVentCmdFault.EN_VENT_FAULT_NONE == Error ...
      | && TRUE != OppositeCmd ...
      | && TRUE != Vent_RecoverDefaultFlag ...
      | && ((FALSE == Vent_CanMessageLostFlag && enProjectType.EN_PROJECT_BM400 == CarType) ...
      | || (enProjectType.EN_PROJECT_BM400 != CarType))]
  data: Level output Enum: enVentLvlSts; StopReason output Enum: enVentStopReason; OriginalLevel input Enum: enVentLvlSts; Error input uint8; CarType input Enum: enProjectType; TRUE parameter; OppositeCmd input uint8; Vent_CanMessageLostFlag input uint8; Vent_RecoverDefaultFlag input uint8; FALSE parameter

== stateflow chart Appl_VentAdj_CtrlModel/UpDataInputInfo/InputSignalProcess/HeatMessage/HeatMessage/OppositeMessageDeal2/OppositeMessageDeal ==
  state HMIMessageDeal [parallel]
    settings: executionOrder=1
    state HMIValid
      en:
      TempHMI = TRUE;
    state HMIInit
      en:
      TempHMI = FALSE;
    (default) -> HMIInit
    HMIInit -> HMIValid : /*档位请求有效*/
        | [(enProjectType.EN_PROJECT_BM400 != CarTypeCfg && (0x1 == HMI_Message || 0x2 == HMI_Message || 0x3 == HMI_Message || 0x5 == HMI_Message)) ...
        | || (enProjectType.EN_PROJECT_BM400 == CarTypeCfg && (0x2 == HMI_Message || 0x3 == HMI_Message || 0x4 == HMI_Message))]
    HMIValid -> HMIInit : /*HMI报文关闭*/
        | [(enProjectType.EN_PROJECT_BM400 != CarTypeCfg && 0x1 != HMI_Message && 0x2 != HMI_Message && 0x3 != HMI_Message&& 0x5 != HMI_Message) ...
        | || (enProjectType.EN_PROJECT_BM400 == CarTypeCfg && 0x2 != HMI_Message && 0x3 != HMI_Message && 0x4 != HMI_Message)]
  state TboxMessageDeal [parallel]
    settings: executionOrder=2
    state TboxValid
      en:
      TempTbox = TRUE;
    state TboxInit
      en:
      TempTbox = FALSE;
    (default) -> TboxMessageDeal.TboxInit
    TboxMessageDeal.TboxInit -> TboxMessageDeal.TboxValid : /*档位请求有效*/
        | [(TRUE == RemoteModeFlag) && (0x1 == Tbox_Message ...
        | || 0x2 == Tbox_Message ...
        | || 0x3 == Tbox_Message)]
    TboxMessageDeal.TboxValid -> TboxMessageDeal.TboxInit : /*Tbox报文关闭*/
        | [0x0 == Tbox_Message || FALSE == RemoteModeFlag]
  state VenStatus [parallel]
    settings: executionOrder=3
    state TboxValid
      en:
      VenSts = TRUE;
    state TboxInit
      en:
      VenSts = FALSE;
    (default) -> VenStatus.TboxInit
    VenStatus.TboxInit -> VenStatus.TboxValid : /* 档位请求有效 且加热配置 */
        | [(TRUE == TempHMI ...
        | || TRUE == TempTbox) && HeatCfg == TRUE]
    VenStatus.TboxValid -> VenStatus.TboxInit : /* 档位请求无效 或加热无配置 */
        | [(FALSE == TempHMI ...
        | && FALSE == TempTbox) || HeatCfg == FALSE]
  data: CarTypeCfg input Enum: enProjectType; RemoteModeFlag input uint8; HMI_Message input uint8; Tbox_Message input uint8; VenSts output uint8; TempHMI local uint8; TRUE parameter; FALSE parameter; TempTbox local uint8; HeatCfg input uint8

== stateflow chart Appl_VentAdj_CtrlModel/LogicCtrl/LocalAdjustCtrl/LimitDeal/TimeoutFunction/Timeout ==
  state Ts = D_HAL_GET_CUR_MS_TS [function]
  state OutTs = TimeDiffTs(lastTs,Ts) [function]
  state TimeCountStatus
    state TimeoutSts
      en:
      Level = InLevel;
      du:
      Level = InLevel;
      ex:
      Timer = 0;
    state Init
      en:
      Level = InLevel;
      Timer = D_HAL_GET_CUR_MS_TS();
      du:
      Level = InLevel;
      ex:
      Timer = D_HAL_GET_CUR_MS_TS();
    (default) -> Init
    Init -> TimeoutSts [order 1] : [TimeDiffTs(Timer,D_HAL_GET_CUR_MS_TS()) >= MaxTime]
        | /TimeoutFlag = TRUE;
    TimeoutSts -> Init : [hasChangedFrom(InLevel,enVentLvlSts.EN_VENT_LVL_OFF)]
    Init -> Init [order 2] : [hasChangedFrom(InLevel,enVentLvlSts.EN_VENT_LVL_OFF)]
  state Default
    en:
    Level = InLevel;
    du:
    Level = InLevel;
  (default) -> Default
  Default -> TimeCountStatus : /*有超时配置
      | && 启动加热&&有时间值 */
      | [TRUE == TimeoutPrm ...
      | && enVentLvlSts.EN_VENT_LVL_OFF != InLevel ...
      | && 0 != MaxTime]
  TimeCountStatus -> Default : /*无超时配置*/
      | [TRUE != TimeoutPrm || 0 == MaxTime]
      | /TimeoutFlag = FALSE;
  data: Ts function_output; lastTs function_input; Ts function_input; OutTs function_output; TimeoutPrm input uint8; TimeoutFlag output uint8; FALSE parameter; TRUE parameter; InLevel input Enum: enVentLvlSts; MaxTime input uint32; Timer local uint32; Level output Enum: enVentLvlSts

== stateflow chart Appl_VentAdj_CtrlModel/LogicCtrl/LocalAdjustCtrl/LimitDeal/TimeoutFunction/Timeout/TimeDiffTs/Chart ==
  (default) -> (junction 3)
  (junction 3) -> (junction 5)
  (junction 5) -> (junction 7) [order 1] : /* 入参比当前大 */
      | [lastTs > Ts]
  (junction 5) -> (junction 13) [order 2] : {OutTs = Ts - lastTs;}
  (junction 7) -> (junction 11) : {OutTs = 0xFFFFFFFF - lastTs + Ts +1;}
  (junction 11) -> (junction 13)
  (junction 13) -> (junction 17)
  data: lastTs input uint32; Ts input uint32; OutTs output uint32

== stateflow chart Appl_VentAdj_CtrlModel/LogicCtrl/LocalAdjustCtrl/VentLevelDeal/LevelAquireFunction2/LevelAquireFunction ==
  state LevelAquire
    (default) -> (junction 92)
    LevelAquire -> (junction 92)
    (junction 92) -> (junction 95) [order 1] : /*加热功能禁能
        | || OFF 电
        | || 发动机不在运行中*/
        | [enVentStopReason.EN_VENT_STOP_R_NONE != DisableSts ...
        | || FALSE == EnableCfg ...
        | || enPowerModeSts.EN_OFF == PowerMode ...
        | || TRUE != EngineSts]
    (junction 92) -> (junction 94) [order 2] : {StopFlag = FALSE;}
    (junction 95) -> (junction 93) : {Level = enVentLvlSts.EN_VENT_LVL_OFF;
        | StopFlag = TRUE;}
    (junction 93) -> (junction 94)
    (junction 94) -> (junction 101)
    (junction 101) -> (junction 21) [order 1] : [StopFlag == FALSE]
    (junction 21) -> (junction 23) [order 1] : [enProjectType.EN_PROJECT_P20 == CarTypeCfg]
    (junction 101) -> (junction 104) [order 2] : {Level = enVentLvlSts.EN_VENT_LVL_OFF;}
    (junction 21) -> (junction 48) [order 2]
    (junction 23) -> (junction 82)
    (junction 82) -> (junction 84) [order 1] : /* 一键开启 且为Hmi控制 */
        | [5 == CAN_Message && Type == 0]
    (junction 82) -> (junction 25) [order 2]
    (junction 84) -> (junction 86) : {Level = CAN_Lvl + 1;}
    (junction 25) -> (junction 27) [order 1] : [4 == CAN_Message]
    (junction 25) -> (junction 29) [order 2] : {TempMsg = CAN_Message + 7;}
    (junction 27) -> (junction 57) : {Level = enVentLvlSts.EN_VENT_LVL_OFF;}
    (junction 48) -> (junction 50) [order 1] : [1 != CAN_Message]
    (junction 48) -> (junction 55) [order 2] : {Level = enVentLvlSts.EN_VENT_LVL_OFF;}
    (junction 50) -> (junction 52) : {TempMsg = CAN_Message;}
    (junction 52) -> (junction 29)
    (junction 29) -> (junction 32) [order 1] : [7 < TempMsg && 11 > TempMsg]
    (junction 29) -> (junction 36) [order 2] : {Level = 0xFF;}
    (junction 32) -> (junction 34)
    (junction 34) -> (junction 38) [order 1] : [8 == TempMsg]
    (junction 34) -> (junction 40) [order 2]
    (junction 38) -> (junction 59) : {Level = enVentLvlSts.EN_VENT_LVL_1;}
    (junction 40) -> (junction 42) [order 1] : [9 == TempMsg]
    (junction 40) -> (junction 46) [order 2] : {Level = enVentLvlSts.EN_VENT_LVL_3;}
    (junction 42) -> (junction 44) : {Level = enVentLvlSts.EN_VENT_LVL_2;}
    (junction 55) -> (junction 104)
    (junction 36) -> (junction 55)
    (junction 46) -> (junction 36)
    (junction 44) -> (junction 46)
    (junction 59) -> (junction 44)
    (junction 57) -> (junction 59)
    (junction 86) -> (junction 57)
    (junction 104) -> (junction 75)
  data: EnableCfg input uint8; CarTypeCfg input Enum: enProjectType; PowerMode input Enum: enPowerModeSts; EngineSts input uint8; CAN_Message input uint8; DisableSts input Enum: enVentStopReason; Level output uint8; TempMsg local uint8; TRUE parameter; FALSE parameter; CAN_Lvl input uint8; Type input; StopFlag local boolean

== stateflow chart Appl_VentAdj_CtrlModel/LogicCtrl/LocalAdjustCtrl/VentLevelDeal/LevelAquireFunction/LevelAquireFunction ==
  state LevelAquire
    (default) -> (junction 92)
    LevelAquire -> (junction 92)
    (junction 92) -> (junction 95) [order 1] : /*加热功能禁能
        | || OFF 电
        | || 发动机不在运行中*/
        | [enVentStopReason.EN_VENT_STOP_R_NONE != DisableSts ...
        | || FALSE == EnableCfg ...
        | || enPowerModeSts.EN_OFF == PowerMode ...
        | || TRUE != EngineSts]
    (junction 92) -> (junction 94) [order 2] : {StopFlag = FALSE;}
    (junction 95) -> (junction 93) : {Level = enVentLvlSts.EN_VENT_LVL_OFF;
        | StopFlag = TRUE;}
    (junction 93) -> (junction 94)
    (junction 94) -> (junction 101)
    (junction 101) -> (junction 21) [order 1] : [StopFlag == FALSE]
    (junction 21) -> (junction 23) [order 1] : [enProjectType.EN_PROJECT_P20 == CarTypeCfg]
    (junction 101) -> (junction 104) [order 2] : {Level = enVentLvlSts.EN_VENT_LVL_OFF;}
    (junction 21) -> (junction 48) [order 2]
    (junction 23) -> (junction 82)
    (junction 82) -> (junction 84) [order 1] : /* 一键开启 且为Hmi控制 */
        | [5 == CAN_Message && Type == 0]
    (junction 82) -> (junction 25) [order 2]
    (junction 84) -> (junction 86) : {Level = CAN_Lvl + 1;}
    (junction 25) -> (junction 27) [order 1] : [4 == CAN_Message]
    (junction 25) -> (junction 29) [order 2] : {TempMsg = CAN_Message + 7;}
    (junction 27) -> (junction 57) : {Level = enVentLvlSts.EN_VENT_LVL_OFF;}
    (junction 48) -> (junction 50) [order 1] : [1 != CAN_Message]
    (junction 48) -> (junction 55) [order 2] : {Level = enVentLvlSts.EN_VENT_LVL_OFF;}
    (junction 50) -> (junction 52) : {TempMsg = CAN_Message;}
    (junction 52) -> (junction 29)
    (junction 29) -> (junction 32) [order 1] : [7 < TempMsg && 11 > TempMsg]
    (junction 29) -> (junction 36) [order 2] : {Level = 0xFF;}
    (junction 32) -> (junction 34)
    (junction 34) -> (junction 38) [order 1] : [8 == TempMsg]
    (junction 34) -> (junction 40) [order 2]
    (junction 38) -> (junction 59) : {Level = enVentLvlSts.EN_VENT_LVL_1;}
    (junction 40) -> (junction 42) [order 1] : [9 == TempMsg]
    (junction 40) -> (junction 46) [order 2] : {Level = enVentLvlSts.EN_VENT_LVL_3;}
    (junction 42) -> (junction 44) : {Level = enVentLvlSts.EN_VENT_LVL_2;}
    (junction 55) -> (junction 104)
    (junction 36) -> (junction 55)
    (junction 46) -> (junction 36)
    (junction 44) -> (junction 46)
    (junction 59) -> (junction 44)
    (junction 57) -> (junction 59)
    (junction 86) -> (junction 57)
    (junction 104) -> (junction 75)
  data: EnableCfg input uint8; CarTypeCfg input Enum: enProjectType; PowerMode input Enum: enPowerModeSts; EngineSts input uint8; CAN_Message input uint8; DisableSts input Enum: enVentStopReason; Level output uint8; TempMsg local uint8; TRUE parameter; FALSE parameter; CAN_Lvl input uint8; Type input; StopFlag local boolean

== stateflow chart Appl_VentAdj_CtrlModel/UpDataInputInfo/InputSignalProcess/VentMessage/VentMessage ==
  state [OutMsgHMI,OutMsgTbox,MixConflictFlg] = MsgConflictFunction2(CarTypeCfg,HMI_Message,Tbox_Message,VentValidFlag) [function]
  state [OutMsgHMI,OutMsgTbox,MixConflictFlg] = MsgConflictFunction1(CarTypeCfg,HMI_Message,Tbox_Message,VentValidFlag) [function]
  state [OutMsgHMI,OutMsgTbox,MixConflictFlg] = MsgConflictFunction(CarTypeCfg,HMI_Message,Tbox_Message,VentValidFlag) [function]
  state Message
    du:
    [DriverHMI_VentMessage,DriverTbox_VentMessage,Driver_MixConflicFlg] = MsgConflictFunction(VentAdj_CarType,VentAdj_DriverHMI_VentMessage,VentAdj_DriverTbox_VentMessage,DriverHeatValid);
    [PassengerHMI_VentMessage,PassengerTbox_VentMessage,Passenger_MixConflicFlg] = MsgConflictFunction1(VentAdj_CarType,VentAdj_PassengerHMI_VentMessage,VentAdj_PassengerTbox_VentMessage,PassengerHeatValid);
    [ThirdHMI_VentMessage,ThirdTbox_VentMessage,Third_MixConflicFlg] = MsgConflictFunction2(VentAdj_CarType,VentAdj_ThirdHMI_VentMessage,VentAdj_ThirdTbox_VentMessage,ThirdHeatValid);
  (default) -> Message
  data: CarTypeCfg function_input; HMI_Message function_input uint8; Tbox_Message function_input uint8; VentValidFlag function_input; OutMsgHMI function_output; OutMsgTbox function_output; MixConflictFlg function_output; CarTypeCfg function_input; HMI_Message function_input uint8; Tbox_Message function_input uint8; VentValidFlag function_input; OutMsgHMI function_output; OutMsgTbox function_output; MixConflictFlg function_output; CarTypeCfg function_input; HMI_Message function_input uint8; Tbox_Message function_input uint8; VentValidFlag function_input; OutMsgHMI function_output; OutMsgTbox function_output; MixConflictFlg function_output; DriverHMI_VentMessage output uint8; DriverTbox_VentMessage output uint8; PassengerHMI_VentMessage output uint8; VentAdj_DriverHMI_VentMessage input; VentAdj_DriverTbox_VentMessage input; VentAdj_PassengerHMI_VentMessage input; VentAdj_PassengerTbox_VentMessage input; VentAdj_ThirdHMI_VentMessage input; VentAdj_ThirdTbox_VentMessage input; DriverHeatValid input; PassengerHeatValid input; ThirdHeatValid input; PassengerTbox_VentMessage output uint8; ThirdHMI_VentMessage output uint8; ThirdTbox_VentMessage output uint8; VentAdj_CarType input; Driver_MixConflicFlg output uint8; Passenger_MixConflicFlg output uint8; Third_MixConflicFlg output uint8

== stateflow chart Appl_VentAdj_CtrlModel/UpDataInputInfo/InputSignalProcess/VentMessage/VentMessage/MsgConflictFunction1/Function ==
  state HMI_MessageDeal [parallel]
    settings: executionOrder=1
    state Default
      en:
      HMI_Flag = FALSE;
    state Valid
      en:
      HMI_Flag = TRUE;
    (default) -> HMI_MessageDeal.Default
    HMI_MessageDeal.Default -> HMI_MessageDeal.Valid : /*HMI通风报文有效0x0:Inactive；0x1:Level 1；1档;0x2:Level 2；2档;0x3:Level 3；3档；0x4:OFF: 0x05 OPEN*/
        | [enVentLvlSts.EN_VENT_LVL_1 == HMI_Message ...
        | || enVentLvlSts.EN_VENT_LVL_2 == HMI_Message ...
        | || enVentLvlSts.EN_VENT_LVL_3 == HMI_Message ...
        | || 4 == HMI_Message || 5 == HMI_Message]
    HMI_MessageDeal.Valid -> HMI_MessageDeal.Default : /*HMI通风报文无效，20240507NXM增加关闭4*/
        | [enVentLvlSts.EN_VENT_LVL_1 != HMI_Message ...
        | && enVentLvlSts.EN_VENT_LVL_2 != HMI_Message ...
        | && enVentLvlSts.EN_VENT_LVL_3 != HMI_Message ...
        | && 4 != HMI_Message && 5 != HMI_Message]
  state Tbox_MessageDeal [parallel]
    settings: executionOrder=2
    state Default
      en:
      Tbox_Flag = FALSE;
    state Valid
      en:
      Tbox_Flag = TRUE;
    (default) -> Tbox_MessageDeal.Default
    Tbox_MessageDeal.Default -> Tbox_MessageDeal.Valid : /*Tbox通风报文有效0x0:No Request；0x1:Heat_1；0x2:Heat_2；0x3:Heat_3；0x4:Close*/
        | [enVentLvlSts.EN_VENT_LVL_1 == Tbox_Message ...
        | || enVentLvlSts.EN_VENT_LVL_2 == Tbox_Message ...
        | || enVentLvlSts.EN_VENT_LVL_3 == Tbox_Message ...
        | || 4 == Tbox_Message]
    Tbox_MessageDeal.Valid -> Tbox_MessageDeal.Default : /*Tbox通风报文无效，20240507NXM增加关闭4*/
        | [enVentLvlSts.EN_VENT_LVL_1 != Tbox_Message ...
        | && enVentLvlSts.EN_VENT_LVL_2 != Tbox_Message ...
        | && enVentLvlSts.EN_VENT_LVL_3 != Tbox_Message ...
        | && 4 != Tbox_Message]
  state MessageConflictDeal [parallel]
    settings: executionOrder=3
    state Default
      en,du:
      OutMsgHMI = HMI_Message;
      OutMsgTbox = Tbox_Message;
      MixConflictFlg = FALSE;
    state VentilateConflict
      en:
      OutMsgHMI = 0;
      OutMsgTbox = 0;
      MixConflictFlg = TRUE;
    state HeatConflict
      en:
      OutMsgHMI = 0;
      OutMsgTbox = 0;
      MixConflictFlg = FALSE;
    (default) -> MessageConflictDeal.Default
    MessageConflictDeal.Default -> VentilateConflict [order 2] : /*通风加热报文同时有效 且非关闭状态 */
        | [FALSE != VentValidFlag ...
        | && ((FALSE != HMI_Flag && 4 != HMI_Message) ...
        | || (FALSE != Tbox_Flag && 4 != Tbox_Message))]
    VentilateConflict -> MessageConflictDeal.Default [order 2] : /*通风加热报文不同时有效 或关闭，20240507NXM修改跳转顺序*/
        | [FALSE == VentValidFlag ...
        | || 4 == HMI_Message ...
        | || 4 == Tbox_Message]
    MessageConflictDeal.Default -> HeatConflict [order 1] : /*P20车型HMI、TBOX通风报文同时有效*/
        | [enProjectType.EN_PROJECT_P20 == CarTypeCfg ...
        | && FALSE != HMI_Flag ...
        | && FALSE != Tbox_Flag]
    HeatConflict -> MessageConflictDeal.Default [order 2] : /*非P20车型||P20车型通风报文不同时有效，20240507NXM*/
        | [enProjectType.EN_PROJECT_P20 != CarTypeCfg ...
        | || (enProjectType.EN_PROJECT_P20 == CarTypeCfg ...
        | && (FALSE == HMI_Flag || FALSE == Tbox_Flag))]
    VentilateConflict -> HeatConflict [order 1] : /*P20车型HMI、TBOX通风报文同时有效*/
        | [enProjectType.EN_PROJECT_P20 == CarTypeCfg ...
        | && FALSE != HMI_Flag ...
        | && FALSE != Tbox_Flag ...
        | && FALSE == VentValidFlag]
    HeatConflict -> VentilateConflict [order 1] : /*通风加热报文同时有效，20240507NXM*/
        | [FALSE != VentValidFlag ...
        | && (FALSE != HMI_Flag ...
        | || FALSE != Tbox_Flag)]
  data: CarTypeCfg input uint8; HMI_Message input; Tbox_Message input; VentValidFlag input uint8; FALSE parameter; OutMsgHMI output uint8; OutMsgTbox output uint8; HMI_Flag local uint8; Tbox_Flag local uint8; TRUE parameter; MixConflictFlg output uint8

== stateflow chart Appl_VentAdj_CtrlModel/LogicCtrl/LocalAdjustCtrl/VentLevelDeal/LevelAquireFunction3/LevelAquireFunction ==
  state LevelAquire
    (default) -> (junction 92)
    LevelAquire -> (junction 92)
    (junction 92) -> (junction 95) [order 1] : /*加热功能禁能
        | || OFF 电
        | || 发动机不在运行中*/
        | [enVentStopReason.EN_VENT_STOP_R_NONE != DisableSts ...
        | || FALSE == EnableCfg ...
        | || enPowerModeSts.EN_OFF == PowerMode ...
        | || TRUE != EngineSts]
    (junction 92) -> (junction 94) [order 2] : {StopFlag = FALSE;}
    (junction 95) -> (junction 93) : {Level = enVentLvlSts.EN_VENT_LVL_OFF;
        | StopFlag = TRUE;}
    (junction 93) -> (junction 94)
    (junction 94) -> (junction 101)
    (junction 101) -> (junction 21) [order 1] : [StopFlag == FALSE]
    (junction 21) -> (junction 23) [order 1] : [enProjectType.EN_PROJECT_P20 == CarTypeCfg]
    (junction 101) -> (junction 104) [order 2] : {Level = enVentLvlSts.EN_VENT_LVL_OFF;}
    (junction 21) -> (junction 48) [order 2]
    (junction 23) -> (junction 82)
    (junction 82) -> (junction 84) [order 1] : /* 一键开启 且为Hmi控制 */
        | [5 == CAN_Message && Type == 0]
    (junction 82) -> (junction 25) [order 2]
    (junction 84) -> (junction 86) : {Level = CAN_Lvl + 1;}
    (junction 25) -> (junction 27) [order 1] : [4 == CAN_Message]
    (junction 25) -> (junction 29) [order 2] : {TempMsg = CAN_Message + 7;}
    (junction 27) -> (junction 57) : {Level = enVentLvlSts.EN_VENT_LVL_OFF;}
    (junction 48) -> (junction 50) [order 1] : [1 != CAN_Message]
    (junction 48) -> (junction 55) [order 2] : {Level = enVentLvlSts.EN_VENT_LVL_OFF;}
    (junction 50) -> (junction 52) : {TempMsg = CAN_Message;}
    (junction 52) -> (junction 29)
    (junction 29) -> (junction 32) [order 1] : [7 < TempMsg && 11 > TempMsg]
    (junction 29) -> (junction 36) [order 2] : {Level = 0xFF;}
    (junction 32) -> (junction 34)
    (junction 34) -> (junction 38) [order 1] : [8 == TempMsg]
    (junction 34) -> (junction 40) [order 2]
    (junction 38) -> (junction 59) : {Level = enVentLvlSts.EN_VENT_LVL_1;}
    (junction 40) -> (junction 42) [order 1] : [9 == TempMsg]
    (junction 40) -> (junction 46) [order 2] : {Level = enVentLvlSts.EN_VENT_LVL_3;}
    (junction 42) -> (junction 44) : {Level = enVentLvlSts.EN_VENT_LVL_2;}
    (junction 55) -> (junction 104)
    (junction 36) -> (junction 55)
    (junction 46) -> (junction 36)
    (junction 44) -> (junction 46)
    (junction 59) -> (junction 44)
    (junction 57) -> (junction 59)
    (junction 86) -> (junction 57)
    (junction 104) -> (junction 75)
  data: EnableCfg input uint8; CarTypeCfg input Enum: enProjectType; PowerMode input Enum: enPowerModeSts; EngineSts input uint8; CAN_Message input uint8; DisableSts input Enum: enVentStopReason; Level output uint8; TempMsg local uint8; TRUE parameter; FALSE parameter; CAN_Lvl input uint8; Type input; StopFlag local boolean
